simulink model "Copy_of_NDI"  (R2024b)
settings: Solver=ode4  StartTime=0  StopTime=100  FixedStep=fcs.Ts  RelTol=1e-3
PreLoadFcn:
  | FlightPhase = 'FallingLeaf';
  | % FlightPhase = 'InAir';
  | % FlightPhase = 'TVC_h10000V617alpha2';
  | run('PreLoadFcn.m')
values from neighbouring files (symbols this model uses):
  ControlAllocation = 1    [PreLoadFcn.m]    (also in RunThis_ChiaWei.m = 4; RunThis_LM.m = 4; RunThis_Shao.m; RunThis_james.m = 10)
  DUmax = IN_MAT(k+4,1:m)'    [LP_def.m]    (also in LP_lift.m; LP_sig.m; LP_thrust.m; PreLoadFcn.m = [Aactuator.right_aileron.RateLimitUpper Aactuator.left_ailer)
  DUmin = IN_MAT(k+5,1:m)'    [LP_def.m]    (also in LP_lift.m; LP_sig.m; LP_thrust.m; PreLoadFcn.m = [Aactuator.right_aileron.RateLimitLower Aactuator.left_ailer)
  g = [ 0  0  32.17 ]    [PreLoadFcn.m]
  hground = 0    [PreLoadFcn.m]
  m = m1-1    [CGIwrap.m]    (also in DAISY_CHAINING.m; DA_Allocation.m; LP_BasicSolution.m; LP_def.m)
  Mode_deflection_aileron = 1    [PreLoadFcn.m]    (also in RunThis_ChiaWei.m; RunThis_Shao.m = 0)
  Mode_deflection_elevator = 1    [PreLoadFcn.m]    (also in RunThis_ChiaWei.m; RunThis_Shao.m = 0)
  Mode_deflection_rudder = 1    [PreLoadFcn.m]    (also in RunThis_ChiaWei.m; RunThis_Shao.m = 0)
  Mode_deflection_TVC_y = 1    [PreLoadFcn.m]    (also in RunThis_ChiaWei.m; RunThis_Shao.m = 2)
  Mode_deflection_TVC_z = 1    [PreLoadFcn.m]    (also in RunThis_ChiaWei.m; RunThis_Shao.m = 0)
  N = IN_MAT(k+7:k+15,1:m)    [CGIwrap.m]    (also in DAISY_CHAINING.m; PreLoadFcn.m = [ 1      0     0.25; RunThis_ChiaWei.m = [ 1      0     0.25; RunThis_LM.m = [ 1      0     0.25)
  Ninv_2nozzle = inv(diag([  1/21.5  1/21.5  1/25  1/25  1/30  1/15  1/15  1/15  1/15 ]))    [PreLoadFcn.m]
  Ninv_no_nozzle = diag([    21.5    21.5    25    25    30    0     0     0     0  ])    [PreLoadFcn.m]
  state0 = [IC.npos IC.epos IC.alt IC.q0 IC.q1 IC.q2 IC.q3  IC.p IC.q IC.r IC.alpha IC.beta IC.mu IC.Vt IC.chi IC.gamma]    [PreLoadFcn.m]
  Umax_2nozzle = [Aactuator.right_aileron.AngleLimitUpper  Aactuator.left_aileron.AngleLimitUpper  Aactuator.right_elevator.AngleLimitUpper Aactuator.left_elevator.AngleLimitUpper  Aactuator.rudder.AngleLimitUpper                  Aactuator.TVC_ry.AngleLimitUpper    Aactuator.TVC_rz.AngleLimitUpper  Aactuator.TVC_ly.AngleLimitUpper    Aactuator.TVC_lz.AngleLimitUpper]    [PreLoadFcn.m]
  Umax_no_nozzle = [Aactuator.right_aileron.AngleLimitUpper  Aactuator.left_aileron.AngleLimitUpper  Aactuator.right_elevator.AngleLimitUpper Aactuator.left_elevator.AngleLimitUpper  Aactuator.rudder.AngleLimitUpper                    0 0 0 0]    [PreLoadFcn.m]
  Umin_2nozzle = [Aactuator.aileron.AngleLimitLower  Aactuator.aileron.AngleLimitLower  Aactuator.elevator.AngleLimitLower Aactuator.elevator.AngleLimitLower  Aactuator.rudder.AngleLimitLower                  Aactuator.TVC_ry.AngleLimitLower    Aactuator.TVC_rz.AngleLimitLower Aactuator.TVC_ly.AngleLimitLower    Aactuator.TVC_lz.AngleLimitLower]    [PreLoadFcn.m]
  Umin_no_nozzle = [Aactuator.right_aileron.AngleLimitLower  Aactuator.left_aileron.AngleLimitLower  Aactuator.right_elevator.AngleLimitLower Aactuator.left_elevator.AngleLimitLower  Aactuator.rudder.AngleLimitLower                    0 0 0 0]    [PreLoadFcn.m]
undefined symbols (not defined in the file or in its folder): Aactuator, ac, AeroCoeff, EngineTable, F, fcs, ft, IC, kg, LandingGear, Light, MIL, PIController, s, Sensor, sigbuilder_block, slug, sysID_DAQ, sysID_OBES, WMM2020
libraries: aerolibconvert2 x31, slpidlib x11, simulink x6, sharedutil x4, aerolibatmos2 x3, aerolibwind2 x3, aerolibbdyn x3, aerolibgravity2 x2, sharedtransform x1
(part 7 of 14)

== system Copy_of_NDI/F-16 Vehicle Systems Model/Vehicle/Propulsion(two_nozzles) ==
  note: Thrust Vector Nozzle Module 向量噴嘴模組
  note: Commands_TVC_ry_pitch_deg
      | Commands_TVC_rz_yaw_deg
      | Commands_TVC_ly_pitch_deg
      | Commands_TVC_lz_yaw_deg
  note: Inlet 進氣道
  note: 高度限制 0 ~ 50000 ft
      | 馬赫數限制 0 ~ 1 馬赫
  note: Thrust Vector Nozzle Module 向量噴嘴模組
  Bus Element In2 : Inport  PortName=fadec_cmd
  In Bus Element3 : Inport  PortName=fadec_cmd  Element=thrust
  In Bus Element1 : Inport  Port=2  PortName=EnvData  Element=Mach
  Bus Element In1 : Inport  Port=3  PortName=PlantData  Element=beta
  Bus Element In : Inport  Port=3  PortName=PlantData  Element=alpha
  In Bus Element : Inport  Port=3  PortName=PlantData  Element=altitude
  Actuators : Subsystem
  Actuators1 : Subsystem
  Add{,1..5} (6 alike) : Sum
  Afterburning Turbofan Jet Engine : Subsystem
  Bus Selector : BusSelector  OutputSignals=TVC_ly_pitch_deg,TVC_lz_yaw_deg
  Bus Selector1 : BusSelector  OutputSignals=TVC_ry_pitch_deg,TVC_rz_yaw_deg
  Cos : Trigonometry  Operator=cos
  Cos1 : Trigonometry  Operator=cos
  Gain1 : Gain  Gain=0.5
  IC1 : InitialCondition  Commented=through  Value=IC.thrust_lbf
  Left Thrust Vector Nozzle ZY : Subsystem
  Mux2 : Mux  Inputs=6
  Product : Product  Inputs=3
  Right Thrust Vector Nozzle ZY : Subsystem
  nozzle position1 : Constant  Value=ac.lt1
  nozzle position2 : Constant  Value=ac.mt
  nozzle position3 : Constant  Value=ac.lt1
  nozzle position4 : Constant  Value=ac.mt
  r2d1 : Gain  Gain=-1  SaturateOnIntegerOverflow=on  OutDataTypeStr=Inherit: Same as input  ParamDataTypeStr=Inherit: Same as input
  FM : Outport
  Bus Element Out : Outport  Port=2  PortName=ActSensor_Out  Element=TVC_ry_pitch_deg
  Bus Element Out1 : Outport  Port=2  PortName=ActSensor_Out  Element=TVC_rz_yaw_deg
  Bus Element Out2 : Outport  Port=2  PortName=ActSensor_Out  Element=TVC_ly_pitch_deg
  Bus Element Out3 : Outport  Port=2  PortName=ActSensor_Out  Element=TVC_lz_yaw_deg
  Bus Element Out4 : Outport  Port=3  PortName=PropData  Element=T
  Bus Element Out5 : Outport  Port=3  PortName=PropData  Element=engine_state
  Bus Element Out15 : Outport  Port=3  PortName=PropData  Element=Tx
  Bus Element Out16 : Outport  Port=3  PortName=PropData  Element=Ty
  Bus Element Out17 : Outport  Port=3  PortName=PropData  Element=Tz
  wires:
  nozzle position1/1 -> Right Thrust Vector Nozzle ZY/3(" lt")
  Product/1 -> Afterburning Turbofan Jet Engine/1(Mach)
  r2d1/1 -> Afterburning Turbofan Jet Engine/2(H (ft))
  Cos/1 -> Product/2
  Bus Element In1/1 -> Cos1/1  "beta (rad)"
  In Bus Element1/1 -> Product/1
  Cos1/1 -> Product/3
  Bus Element In/1 -> Cos/1  "alpha (rad)"
  In Bus Element/1 -> r2d1/1
  Bus Element In2/1 -> Actuators1/1(Commands), Actuators/1(Commands)
  Right Thrust Vector Nozzle ZY/1(Trx) -> Add/1
  Right Thrust Vector Nozzle ZY/2(Try) -> Add1/1
  Right Thrust Vector Nozzle ZY/3(Trz) -> Add2/1
  nozzle position2/1 -> Right Thrust Vector Nozzle ZY/4(" mt")
  IC1/1 -> Gain1/1, Bus Element Out4/1
  Afterburning Turbofan Jet Engine/1(T (lbf)) -> IC1/1  "thrust"
  Afterburning Turbofan Jet Engine/2(engine_state) -> Bus Element Out5/1
  In Bus Element3/1 -> Afterburning Turbofan Jet Engine/3(Tc (lbf))  "Commands_Tc"
  Gain1/1 -> Left Thrust Vector Nozzle ZY/1(T), Right Thrust Vector Nozzle ZY/1(T)
  Right Thrust Vector Nozzle ZY/4(Mrx) -> Add3/1
  Right Thrust Vector Nozzle ZY/5(Mry) -> Add4/1
  Right Thrust Vector Nozzle ZY/6(Mrz) -> Add5/1
  nozzle position3/1 -> Left Thrust Vector Nozzle ZY/3(" lt")
  nozzle position4/1 -> Left Thrust Vector Nozzle ZY/4(" mt")
  Actuators1/1(ActPositions) -> Left Thrust Vector Nozzle ZY/2(Actuator (deg))
  Left Thrust Vector Nozzle ZY/1(Tlx) -> Add/2
  Left Thrust Vector Nozzle ZY/2(Tly) -> Add1/2
  Left Thrust Vector Nozzle ZY/3(Tlz) -> Add2/2
  Left Thrust Vector Nozzle ZY/4(Mlx) -> Add3/2
  Left Thrust Vector Nozzle ZY/5(Mly) -> Add4/2
  Left Thrust Vector Nozzle ZY/6(Mlz) -> Add5/2
  Add/1 -> Bus Element Out15/1, Mux2/1
  Add1/1 -> Bus Element Out16/1, Mux2/2
  Add2/1 -> Mux2/3, Bus Element Out17/1
  Add3/1 -> Mux2/4
  Add4/1 -> Mux2/5
  Add5/1 -> Mux2/6
  Mux2/1 -> FM/1
  Actuators/2(ActSensor_Out) -> Bus Selector1/1
  Actuators1/2(ActSensor_Out) -> Bus Selector/1
  Bus Selector/1 -> Bus Element Out2/1  "<TVC_ly_pitch_deg>"
  Bus Selector/2 -> Bus Element Out3/1  "<TVC_lz_yaw_deg>"
  Bus Selector1/1 -> Bus Element Out/1  "<TVC_ry_pitch_deg>"
  Bus Selector1/2 -> Bus Element Out1/1  "<TVC_rz_yaw_deg>"
  Actuators/1(ActPositions) -> Right Thrust Vector Nozzle ZY/2(Actuator (deg))

== system Copy_of_NDI/F-16 Vehicle Systems Model/pqr NDI Controller/Control Allocation ==
  note: 多級偽逆法
  note: 108、109年度學合案
      | 2019張舜淵論文配置法
  note: 最小雷達散射截面積
  note: 最小控制面偏轉量
  note: 最小向量推力
  note: 最大升力
  note: 線性規劃法基礎解
  note: 管理方案三：廣義逆類配置法
  note: 管理方案二：基於期望力矩
  note: 直接幾何法
  note: 多級偽逆法
  note: 串接鏈配置法
  note: 加權偽逆法
  IN_MAT1 : Inport
  alpha (deg) : Inport  Port=2
  Vt (ft/s) : Inport  Port=3
  altitude (ft) : Inport  Port=4
  y_bar : Inport  Port=5
  g1 : Inport  Port=6
  N : Inport  Port=7
  Abs : Abs  SaturateOnIntegerOverflow=off
  Abs1 : Abs  SaturateOnIntegerOverflow=off
  Abs2 : Abs  SaturateOnIntegerOverflow=off
  CGIwrap : Subsystem  TreatAsAtomicUnit=on
  CGIwrap1 : Subsystem  TreatAsAtomicUnit=on
  Chart : Stateflow chart  TreatAsAtomicUnit=on  SystemSampleTime=fcs.Ts
      settings: PortSchema="{\"entries\":[{\"content\":{\"sides\":[{\"content\":{\"connectorIds\":[\"In6\",\"In1\",\"In2\",\"In4\",\"In3\",\"In5\"]},\"type\":\"ConnectorPlacement.EquallySpacedRectSide\",\"uuid\":\"6d076ae3-a9f2-4680-9177-aea4e2fc761d\"},{\"content\":{\"connectorIds\":[\"Out1\"],\"side\":\"RIGHT\"},\"type\":\"ConnectorPlacement.EquallySpacedRectSide\",\"uuid\":\"02bbf86f-ce68-419e-b070-bdc8bcbcb5dc\"},{\"content\":{\"connectorIds\":[],\"side\":\"TOP\"},\"type\":\"ConnectorPlacement.EquallySpacedRectSide\",\"uuid\":\"3dbba490-ab37-41e3-b3e5-776a7fc0e7cf\"}]},\"type\":\"ConnectorPlacement.EquallySpacedConnector\",\"uuid\":\"e8ffa1d9-13bd-4b1f-b66c-de77a24e235e\"}],\"packageUris\":[\"http://schema.mathworks.com/mf0/Connector/19700101\"],\"version\":\"1.0\"}"
  Constant : Constant  Value=0
  ControlAllocation : Constant  Value=ControlAllocation
  DAISY_CHAINING : Subsystem  TreatAsAtomicUnit=on
  DA_Allocation : Subsystem  TreatAsAtomicUnit=on
  Discrete Derivative : simulink/Discrete/Discrete Derivative  gainval=1.0  ICPrevScaledInput=0.0  OutMin=[]  OutMax=[]  OutDataType=fixdt(1, 16)  OutScaling=2^-10  DoSatur=off
  Discrete Derivative1 : simulink/Discrete/Discrete Derivative  gainval=1.0  ICPrevScaledInput=0.0  OutMin=[]  OutMax=[]  OutDataType=fixdt(1, 16)  OutScaling=2^-10  DoSatur=off
  IC : InitialCondition  Value=0
  IC1 : InitialCondition  Value=0
  IC2 : InitialCondition  Value=[0 0 0 0 0 0 0 0 0]
  If : If  IfExpression=u1 == 1  ElseIfExpressions=u1 == 2,u1 == 3,u1 == 4,u1 == 5,u1==6,u1==7,u1==8,u1==9,u1==10,u1==11,u1==12
  LP_BasicSolution : Subsystem  TreatAsAtomicUnit=on
  LP_def : Subsystem  TreatAsAtomicUnit=on
  LP_lift : Subsystem  TreatAsAtomicUnit=on
  LP_sig : Subsystem  TreatAsAtomicUnit=on
  LP_thrust : Subsystem  TreatAsAtomicUnit=on
  Manual Switch : ManualSwitch  CurrentSetting=0
  Merge1 : Merge  Inputs=13
  Pseudo_inverses_ShunYuanChang2019 : Subsystem  TreatAsAtomicUnit=on
  To Workspace : ToWorkspace  VariableName=u  SaveFormat=Timeseries  SampleTime=-1
  To Workspace1 : ToWorkspace  VariableName=altitude_dot  SaveFormat=Timeseries  SampleTime=-1
  To Workspace2 : ToWorkspace  VariableName=Vt_dot  SaveFormat=Timeseries  SampleTime=-1
  Weighted_Pseudo_inverses : Subsystem  TreatAsAtomicUnit=on
  control_management2 : Subsystem  TreatAsAtomicUnit=on
  control_management3 : Subsystem  TreatAsAtomicUnit=on
  Du : Outport
  wires:
  DAISY_CHAINING/1(Out1) -> Merge1/2
  Weighted_Pseudo_inverses/1(Out1) -> Merge1/1
  IN_MAT1/1 -> LP_thrust/1(IN_MAT), LP_sig/1(IN_MAT), CGIwrap1/1(IN_MAT), LP_def/1(IN_MAT), LP_lift/1(IN_MAT), control_management2/1(IN_MAT), DA_Allocation/1(IN_MAT), CGIwrap/1(IN_MAT), Weighted_Pseudo_inverses/1(IN_MAT), DAISY_CHAINING/1(IN_MAT), control_management3/1(IN_MAT), LP_BasicSolution/1(IN_MAT)
  Chart/1(CA) -> Manual Switch/1
  ControlAllocation/1 -> Manual Switch/2
  LP_thrust/1(Out1) -> Merge1/9
  LP_def/1(Out1) -> Merge1/10
  LP_sig/1(Out1) -> Merge1/11
  alpha (deg)/1 -> Chart/1(alpha)
  altitude (ft)/1 -> Abs/1
  Abs/1 -> Chart/3(altitude), Discrete Derivative1/1
  Discrete Derivative/1 -> Abs1/1
  Discrete Derivative1/1 -> Abs2/1
  Vt (ft/s)/1 -> Chart/2(Vt), Discrete Derivative/1
  IC/1 -> Chart/5(altitude_dot), To Workspace1/1
  Abs2/1 -> IC/1
  Abs1/1 -> IC1/1
  IC1/1 -> Chart/4(Vt_dot), To Workspace2/1
  Pseudo_inverses_ShunYuanChang2019/1(Output) -> Merge1/12
  y_bar/1 -> Pseudo_inverses_ShunYuanChang2019/1(y_bar)
  g1/1 -> Pseudo_inverses_ShunYuanChang2019/2(g1)
  N/1 -> Pseudo_inverses_ShunYuanChang2019/3(N)
  Constant/1 -> Chart/6(switchhh)
  LP_lift/1(Out1) -> Merge1/8
  IC2/1 -> Du/1
  Merge1/1 -> IC2/1
  Manual Switch/1 -> If/1, To Workspace/1
  CGIwrap1/1(Out1) -> Merge1/13
  DA_Allocation/1(Out1) -> Merge1/4
  CGIwrap/1(Out1) -> Merge1/3
  LP_BasicSolution/1(Out1) -> Merge1/7
  control_management3/1(Out1) -> Merge1/6
  control_management2/1(Out1) -> Merge1/5
  If/1 -> Weighted_Pseudo_inverses/Action
  If/2 -> DAISY_CHAINING/Action
  If/3 -> CGIwrap/Action
  If/4 -> DA_Allocation/Action
  If/5 -> control_management2/Action
  If/6 -> control_management3/Action
  If/7 -> LP_BasicSolution/Action
  If/8 -> LP_lift/Action
  If/9 -> LP_thrust/Action
  If/10 -> LP_def/Action
  If/11 -> LP_sig/Action
  If/12 -> Pseudo_inverses_ShunYuanChang2019/Action
  If/13 -> CGIwrap1/Action

== system Copy_of_NDI/F-16 Vehicle Systems Model/pqr NDI Controller/MakeINMAT ==
  note: 飛控系統的取樣時間(秒)
  note: 控制配置的權重矩陣 $N^{-1}$
      | (定義於 PreLoadFcn.m)
  note: 下標1表示在列後面擴增
      | 下標2表示在行後面擴增
  f1 : Inport
  g1 : Inport  Port=2
  In3 : Inport  Port=3
  Constant1 : Constant  Value=[0;0;0;0;0]
  Constant10 : Constant  Value=Umin_no_nozzle
  Constant2 : Constant  Value=Umax_2nozzle
  Constant3 : Constant  Value=Umin_2nozzle
  Constant4 : Constant  Value=[1 1 1 1 1 1 1 1 1]
  Constant5 : Constant  Value=fcs.Ts
  Constant6 : Constant  Value=DUmax
  Constant7 : Constant  Value=[0;0;0;0;0;0;0;0;0]
  Constant8 : Constant  Value=DUmin
  Constant9 : Constant  Value=Umax_no_nozzle
  Manual Switch : ManualSwitch
  Manual Switch1 : ManualSwitch
  Manual Switch2 : ManualSwitch
  Matrix Concatenate{,2,4,6} (4 alike) : Concatenate  Mode=Multidimensional array  ConcatenateDimension=2
  Matrix Concatenate3 : Concatenate  NumInputs=5  Mode=Multidimensional array
  Matrix Concatenate5 : Concatenate  NumInputs=4  Mode=Multidimensional array
  Signal Specification : SignalSpecification  Dimensions=[3 1]
  Signal Specification{1..2,4..9} (8 alike) : SignalSpecification  Dimensions=[1,9]
  Signal Specification3 : SignalSpecification  Dimensions=[3 9]
  To Workspace2 : ToWorkspace  VariableName=B_matrix  SaveFormat=Timeseries  SampleTime=-1
  inverse of weighting matrix N : Constant  Value=Ninv_2nozzle
  inverse of weighting matrix N1 : Constant  Value=Ninv_no_nozzle
  IN_MAT : Outport
  wires:
  Matrix Concatenate6/1 -> Matrix Concatenate5/4
  Matrix Concatenate3/1 -> Matrix Concatenate4/1
  Signal Specification3/1 -> Matrix Concatenate/1
  Manual Switch1/1 -> Matrix Concatenate3/2
  Matrix Concatenate4/1 -> Matrix Concatenate5/3
  Matrix Concatenate/1 -> Matrix Concatenate5/1
  Signal Specification/1 -> Matrix Concatenate/2
  Manual Switch/1 -> Matrix Concatenate3/1
  Matrix Concatenate5/1 -> IN_MAT/1
  f1/1 -> Signal Specification/1
  g1/1 -> To Workspace2/1, Signal Specification3/1
  Constant4/1 -> Signal Specification4/1
  Signal Specification4/1 -> Matrix Concatenate3/5
  Constant1/1 -> Matrix Concatenate4/2
  In3/1 -> Signal Specification5/1
  Signal Specification5/1 -> Matrix Concatenate2/1
  Constant5/1 -> Matrix Concatenate2/2
  Matrix Concatenate2/1 -> Matrix Concatenate5/2
  Signal Specification6/1 -> Matrix Concatenate3/3
  Signal Specification7/1 -> Matrix Concatenate3/4
  Constant6/1 -> Signal Specification6/1  "Umax"
  Constant8/1 -> Signal Specification7/1  "Umax"
  Constant3/1 -> Signal Specification2/1  "Umin"
  Constant2/1 -> Signal Specification1/1  "Umax"
  Signal Specification1/1 -> Manual Switch/1
  Signal Specification2/1 -> Manual Switch1/1
  Signal Specification8/1 -> Manual Switch/2
  Constant9/1 -> Signal Specification8/1  "Umax"
  Signal Specification9/1 -> Manual Switch1/2
  Constant10/1 -> Signal Specification9/1  "Umin"
  Constant7/1 -> Matrix Concatenate6/2
  inverse of weighting matrix N/1 -> Manual Switch2/1
  inverse of weighting matrix N1/1 -> Manual Switch2/2
  Manual Switch2/1 -> Matrix Concatenate6/1

== system Copy_of_NDI/F-16 Vehicle Systems Model/pqr NDI Controller/Mode_deflection ==
  note: 偏轉模式： 0=傳統左右副翼差動
      | 1=左右副翼獨立偏轉
      | 其它=左右副翼獨立偏轉
  note: 偏轉模式： 0=傳統左右升降舵同動
      | 1=左右升降舵獨立偏轉
      | 其它=左右升降舵獨立偏轉
  note: 偏轉模式： 0=傳統左右方向舵同動
      | 1=左右方向舵獨立偏轉
      | 2=左右方向舵差動(產生減速效果)
      | 其它=左右方向舵獨立偏轉
  note: 偏轉模式： 0=傳統左右向量噴嘴固定不動
      | 1=左右向量噴嘴左右獨立偏轉
      | 2=左右向量噴嘴左右同動
      | 其它=左右向量噴嘴左右獨立偏轉
  note: 偏轉模式： 0=傳統左右向量噴嘴固定不動
      | 1=左右向量噴嘴上下獨立偏轉
      | 2=左右向量噴嘴上下同動(產生俯仰)
      | 3=左右向量噴嘴上下差動(產生滾轉)
      | 其它=左右向量噴嘴上下獨立偏轉
  dra : Inport
  dla : Inport  Port=2
  dre : Inport  Port=3
  dle : Inport  Port=4
  drr : Inport  Port=5
  dlr : Inport  Port=6
  dry : Inport  Port=7
  drz : Inport  Port=8
  dly : Inport  Port=9
  dlz : Inport  Port=10
  Constant{,3,7,10} (4 alike) : Constant  Value=0
  Constant1 : Constant  Value=Mode_deflection_aileron
  Constant2 : Constant  Value=Mode_deflection_elevator
  Constant4 : Constant  Value=Mode_deflection_TVC_y
  Constant5 : Constant  Value=Mode_deflection_rudder
  Constant6 : Constant  Value=Mode_deflection_TVC_y
  Constant8 : Constant  Value=Mode_deflection_TVC_z
  Constant9 : Constant  Value=Mode_deflection_TVC_z
  Gain : Gain  Gain=-1
  Gain1 : Gain  Gain=-1
  Gain2 : Gain  Gain=-1
  Multiport Switch : MultiPortSwitch  DataPortOrder=Zero-based contiguous  Inputs=2  zeroidx=on  SaturateOnIntegerOverflow=off  InputSameDT=off
  Multiport Switch1 : MultiPortSwitch  DataPortOrder=Zero-based contiguous  Inputs=2  zeroidx=on  SaturateOnIntegerOverflow=off  InputSameDT=off
  Multiport Switch2 : MultiPortSwitch  DataPortOrder=Zero-based contiguous  DataPortForDefault=Additional data port  zeroidx=on  SaturateOnIntegerOverflow=off  InputSameDT=off
  Multiport Switch3 : MultiPortSwitch  DataPortOrder=Zero-based contiguous  Inputs=4  DataPortForDefault=Additional data port  zeroidx=on  SaturateOnIntegerOverflow=off  InputSameDT=off
  Multiport Switch4 : MultiPortSwitch  DataPortOrder=Zero-based contiguous  DataPortForDefault=Additional data port  zeroidx=on  SaturateOnIntegerOverflow=off  InputSameDT=off
  Multiport Switch5 : MultiPortSwitch  DataPortOrder=Zero-based contiguous  Inputs=4  DataPortForDefault=Additional data port  zeroidx=on  SaturateOnIntegerOverflow=off  InputSameDT=off
  Multiport Switch6 : MultiPortSwitch  DataPortOrder=Zero-based contiguous  DataPortForDefault=Additional data port  zeroidx=on  SaturateOnIntegerOverflow=off  InputSameDT=off
  right_aileron : Outport  VectorParamsAs1DForOutWhenUnconnected=off
  left_aileron : Outport  Port=2  VectorParamsAs1DForOutWhenUnconnected=off
  right_elevator : Outport  Port=3  VectorParamsAs1DForOutWhenUnconnected=off
  left_elevator : Outport  Port=4  VectorParamsAs1DForOutWhenUnconnected=off
  rudder : Outport  Port=5  VectorParamsAs1DForOutWhenUnconnected=off
  left_rudder : Outport  Port=6  VectorParamsAs1DForOutWhenUnconnected=off
  "TVC_ry " : Outport  Port=7  VectorParamsAs1DForOutWhenUnconnected=off
  TVC_rz : Outport  Port=8  VectorParamsAs1DForOutWhenUnconnected=off
  "TVC_ly " : Outport  Port=9  VectorParamsAs1DForOutWhenUnconnected=off
  "TVC_lz " : Outport  Port=10  VectorParamsAs1DForOutWhenUnconnected=off
  wires:
  Gain2/1 -> Multiport Switch3/5
  Gain1/1 -> Multiport Switch4/4
  Multiport Switch4/1 -> left_rudder/1
  Multiport Switch2/1 -> "TVC_lz "/1
  Constant3/1 -> Multiport Switch2/2
  drz/1 -> Multiport Switch6/3, Multiport Switch6/4, Multiport Switch6/5, Multiport Switch2/4
  Constant10/1 -> Multiport Switch6/2
  Multiport Switch6/1 -> TVC_rz/1
  Constant8/1 -> Multiport Switch2/1
  dlz/1 -> Multiport Switch2/3, Multiport Switch2/5
  Constant9/1 -> Multiport Switch6/1
  Multiport Switch5/1 -> "TVC_ry "/1
  Constant7/1 -> Multiport Switch5/2
  Constant6/1 -> Multiport Switch5/1
  Constant/1 -> Multiport Switch3/2
  dly/1 -> Multiport Switch3/6, Multiport Switch3/3
  Multiport Switch/1 -> left_aileron/1
  dre/1 -> right_elevator/1, Multiport Switch1/2
  dle/1 -> Multiport Switch1/3
  Multiport Switch1/1 -> left_elevator/1
  dla/1 -> Multiport Switch/3
  drr/1 -> Multiport Switch4/2, Gain1/1, rudder/1
  dry/1 -> Gain2/1, Multiport Switch3/4, Multiport Switch5/6, Multiport Switch5/5, Multiport Switch5/4, Multiport Switch5/3
  Constant5/1 -> Multiport Switch4/1
  dra/1 -> right_aileron/1, Gain/1
  Constant2/1 -> Multiport Switch1/1
  Constant4/1 -> Multiport Switch3/1
  Gain/1 -> Multiport Switch/2
  Constant1/1 -> Multiport Switch/1
  dlr/1 -> Multiport Switch4/3, Multiport Switch4/5
  Multiport Switch3/1 -> "TVC_ly "/1

== system Copy_of_NDI/F-16 Vehicle Systems Model/pqr NDI Controller/control matrix g1 ==
  note: m
      | ix
      | iy
      | iz
      | ixy
      | ixz
      | iyz
  note: 1  gp_dra1
      |     gp_dla1
      |     gp_dre1
      |     gp_dle1
      |     gp_dr1
      |     gp_dra2
      |     gp_dla2
      |     gp_dre2
      |     gp_dle2
      |     gp_dr2
      |
      | 11 gq_dra
      |      gq_dla
      |      gq_dre
      |      gq_dle
      |
      | 15 gr_dra1
      |      gr_dla1
      |      gr_dre1
      |      gr_dle1
      |      gr_dr1
      |      gr_dra2
      |      gr_dla2
      |      gr_dre2
      |      gr_dle2
      |      gr_dr2
  note: $g_1 {\left({\overset{-}{x} }_1 \right)}={\left[\begin{array}{ccccccccc} g_{p_{\delta_{ra} } } & g_{p_{\delta_{la} } } & g_{p_{\delta_{re} } } & g_{p_{\delta_{le} } } & g_{p_{\delta_r } } & g_{p_{\delta_{ry} } } & g_{p_{\delta_{rz} } } & g_{p_{\delta_{ly} } } & g_{p_{\delta_{lz} } } \\ g_{q_{\delta_{ra} } } & g_{q_{\delta_{la} } } & g_{q_{\delta_{re} } } & g_{q_{\delta_{le} } } & 0 & g_{q_{\delta_{ry} } } & 0 & g_{q_{\delta_{ly} } } & 0 \\ g_{r_{\delta_{ra} } } & g_{r_{\delta_{la} } } & g_{r_{\delta_{re} } } & g_{r_{\delta_{le} } } & g_{r_{\delta_r } } & g_{r_{\delta_{ry} } } & g_{r_{\delta_{rz} } } & g_{r_{\delta_{ly} } } & g_{r_{\delta_{lz} } } \end{array}\right]}$
  coef g : Inport
  Thrust T : Inport  Port=2
  Engine nozzle after of c.g.1 : Constant  Value=ac.lt1
  Engine nozzle after of c.g.2 : Constant  Value=ac.mt
  Gain : Gain  Gain=1/2
  Ix(slug*ft^2) : Constant  Value=ac.Ix
  Ixy(slug*ft^2) : Constant  Value=ac.Ixy
  Ixz(slug*ft^2) : Constant  Value=ac.Ixz
  Iy(slug*ft^2) : Constant  Value=ac.Iy
  Iyz(slug*ft^2) : Constant  Value=ac.Iyz
  Iz(slug*ft^2) : Constant  Value=ac.Iz
  Matrix Concatenate : Concatenate  NumInputs=3  Mode=Multidimensional array
  Mux : Mux  Inputs=7
  "Pitching " : Subsystem
  "Rolling " : Subsystem
  "Yawing " : Subsystem
  m(slugs) : Constant  Value=ac.m
  g1 : Outport  VectorParamsAs1DForOutWhenUnconnected=off
  wires:
  "Yawing "/1(g1 Row3) -> Matrix Concatenate/3
  "Pitching "/1(g1 Row2) -> Matrix Concatenate/2
  "Rolling "/1(g1 Row1) -> Matrix Concatenate/1
  Mux/1 -> "Rolling "/2(inertia), "Pitching "/2(inertia), "Yawing "/2(inertia)
  coef g/1 -> "Yawing "/1(control_g), "Pitching "/1(control_g), "Rolling "/1(control_g)
  Thrust T/1 -> Gain/1
  Engine nozzle after of c.g.1/1 -> "Yawing "/4("lt1 "), "Pitching "/4(lt1), "Rolling "/4(lt1)
  Iyz(slug*ft^2)/1 -> Mux/7
  Ix(slug*ft^2)/1 -> Mux/2
  Iy(slug*ft^2)/1 -> Mux/3
  Ixy(slug*ft^2)/1 -> Mux/5
  Ixz(slug*ft^2)/1 -> Mux/6
  Iz(slug*ft^2)/1 -> Mux/4
  m(slugs)/1 -> Mux/1
  Matrix Concatenate/1 -> g1/1
  Engine nozzle after of c.g.2/1 -> "Rolling "/5(mt), "Pitching "/5(mt), "Yawing "/5(mt)
  Gain/1 -> "Rolling "/3(Thrust), "Pitching "/3(Thrust), "Yawing "/3(Thrust)

== system Copy_of_NDI/F-16 Vehicle Systems Model/sysID_Onboard_Excitation_System/Mode_deflection ==
  note: 偏轉模式： 0=傳統左右副翼差動
      | 1=左右副翼獨立偏轉
      | 其它=左右副翼獨立偏轉
  note: 偏轉模式： 0=傳統左右升降舵同動
      | 1=左右升降舵獨立偏轉
      | 其它=左右升降舵獨立偏轉
  note: 偏轉模式： 0=傳統左右方向舵同動
      | 1=左右方向舵獨立偏轉
      | 2=左右方向舵差動(產生減速效果)
      | 其它=左右方向舵獨立偏轉
  note: 偏轉模式： 0=傳統左右向量噴嘴固定不動
      | 1=左右向量噴嘴左右獨立偏轉
      | 2=左右向量噴嘴左右同動
      | 其它=左右向量噴嘴左右獨立偏轉
  note: 偏轉模式： 0=傳統左右向量噴嘴固定不動
      | 1=左右向量噴嘴上下獨立偏轉
      | 2=左右向量噴嘴上下同動(產生俯仰)
      | 3=左右向量噴嘴上下差動(產生滾轉)
      | 其它=左右向量噴嘴上下獨立偏轉
  dra : Inport
  dla : Inport  Port=2
  dre : Inport  Port=3
  dle : Inport  Port=4
  drr : Inport  Port=5
  dlr : Inport  Port=6
  dry : Inport  Port=7
  drz : Inport  Port=8
  dly : Inport  Port=9
  dlz : Inport  Port=10
  Constant{,3,7,10} (4 alike) : Constant  Value=0
  Constant1 : Constant  Value=Mode_deflection_aileron
  Constant2 : Constant  Value=Mode_deflection_elevator
  Constant4 : Constant  Value=Mode_deflection_TVC_y
  Constant5 : Constant  Value=Mode_deflection_rudder
  Constant6 : Constant  Value=Mode_deflection_TVC_y
  Constant8 : Constant  Value=Mode_deflection_TVC_z
  Constant9 : Constant  Value=Mode_deflection_TVC_z
  Gain : Gain  Gain=-1
  Gain1 : Gain  Gain=-1
  Gain2 : Gain  Gain=-1
  Multiport Switch : MultiPortSwitch  DataPortOrder=Zero-based contiguous  Inputs=2  zeroidx=on  SaturateOnIntegerOverflow=off  InputSameDT=off
  Multiport Switch1 : MultiPortSwitch  DataPortOrder=Zero-based contiguous  Inputs=2  zeroidx=on  SaturateOnIntegerOverflow=off  InputSameDT=off
  Multiport Switch2 : MultiPortSwitch  DataPortOrder=Zero-based contiguous  DataPortForDefault=Additional data port  zeroidx=on  SaturateOnIntegerOverflow=off  InputSameDT=off
  Multiport Switch3 : MultiPortSwitch  DataPortOrder=Zero-based contiguous  Inputs=4  DataPortForDefault=Additional data port  zeroidx=on  SaturateOnIntegerOverflow=off  InputSameDT=off
  Multiport Switch4 : MultiPortSwitch  DataPortOrder=Zero-based contiguous  DataPortForDefault=Additional data port  zeroidx=on  SaturateOnIntegerOverflow=off  InputSameDT=off
  Multiport Switch5 : MultiPortSwitch  DataPortOrder=Zero-based contiguous  Inputs=4  DataPortForDefault=Additional data port  zeroidx=on  SaturateOnIntegerOverflow=off  InputSameDT=off
  Multiport Switch6 : MultiPortSwitch  DataPortOrder=Zero-based contiguous  DataPortForDefault=Additional data port  zeroidx=on  SaturateOnIntegerOverflow=off  InputSameDT=off
  right_aileron : Outport  VectorParamsAs1DForOutWhenUnconnected=off
  left_aileron : Outport  Port=2  VectorParamsAs1DForOutWhenUnconnected=off
  right_elevator : Outport  Port=3  VectorParamsAs1DForOutWhenUnconnected=off
  left_elevator : Outport  Port=4  VectorParamsAs1DForOutWhenUnconnected=off
  rudder : Outport  Port=5  VectorParamsAs1DForOutWhenUnconnected=off
  left_rudder : Outport  Port=6  VectorParamsAs1DForOutWhenUnconnected=off
  "TVC_ry " : Outport  Port=7  VectorParamsAs1DForOutWhenUnconnected=off
  TVC_rz : Outport  Port=8  VectorParamsAs1DForOutWhenUnconnected=off
  "TVC_ly " : Outport  Port=9  VectorParamsAs1DForOutWhenUnconnected=off
  "TVC_lz " : Outport  Port=10  VectorParamsAs1DForOutWhenUnconnected=off
  wires:
  Gain2/1 -> Multiport Switch3/5
  Gain1/1 -> Multiport Switch4/4
  Multiport Switch4/1 -> left_rudder/1
  Multiport Switch2/1 -> "TVC_lz "/1
  Constant3/1 -> Multiport Switch2/2
  drz/1 -> Multiport Switch6/3, Multiport Switch6/4, Multiport Switch6/5, Multiport Switch2/4
  Constant10/1 -> Multiport Switch6/2
  Multiport Switch6/1 -> TVC_rz/1
  Constant8/1 -> Multiport Switch2/1
  dlz/1 -> Multiport Switch2/3, Multiport Switch2/5
  Constant9/1 -> Multiport Switch6/1
  Multiport Switch5/1 -> "TVC_ry "/1
  Constant7/1 -> Multiport Switch5/2
  Constant6/1 -> Multiport Switch5/1
  Constant/1 -> Multiport Switch3/2
  dly/1 -> Multiport Switch3/6, Multiport Switch3/3
  Multiport Switch/1 -> left_aileron/1
  dre/1 -> right_elevator/1, Multiport Switch1/2
  dle/1 -> Multiport Switch1/3
  Multiport Switch1/1 -> left_elevator/1
  dla/1 -> Multiport Switch/3
  drr/1 -> Multiport Switch4/2, Gain1/1, rudder/1
  dry/1 -> Gain2/1, Multiport Switch3/4, Multiport Switch5/6, Multiport Switch5/5, Multiport Switch5/4, Multiport Switch5/3
  Constant5/1 -> Multiport Switch4/1
  dra/1 -> right_aileron/1, Gain/1
  Constant2/1 -> Multiport Switch1/1
  Constant4/1 -> Multiport Switch3/1
  Gain/1 -> Multiport Switch/2
  Constant1/1 -> Multiport Switch/1
  dlr/1 -> Multiport Switch4/3, Multiport Switch4/5
  Multiport Switch3/1 -> "TVC_ly "/1

== system Copy_of_NDI/F-16 Vehicle Systems Model/sysID_Onboard_Excitation_System/signal generator ==
  note: ROM記憶體的指標(Pointer)
  note: 唯讀記憶體，裡面存放波形
  isTurnOn : Inport
  Enable : Inport  Port=2
  sysID_isDone : Inport  Port=3
  Constant1 : Constant  Value=sysID_OBES.TVC_ry.amplitude
  Index Vector : MultiPortSwitch  Inputs=1  SaturateOnIntegerOverflow=off  InputSameDT=off
  Logical Operator1 : Logic  AllPortsSameDT=off  OutDataTypeStr=boolean
  Logical Operator3 : Logic  Operator=NOT  AllPortsSameDT=off  OutDataTypeStr=boolean
  Logical Operator4 : Logic  AllPortsSameDT=off  OutDataTypeStr=boolean
  Pause Counter : Subsystem  TreatAsAtomicUnit=on
  Product : Product
  ROM : Constant  Value=sysID_OBES.TVC_ry.wave
  TVC_ry_delay : Delay  DelayLength=sysID_OBES.TVC_ry.delay/sysID_OBES.Ts  SampleTime=sysID_OBES.Ts
  signal : Outport  OutputWhenDisabled=reset  InitialOutput=0
  isDone : Outport  Port=2
  wires:
  ROM/1 -> Index Vector/2
  Pause Counter/1(CountValue) -> Index Vector/1  "Pointer"
  Pause Counter/2(isCountDone) -> isDone/1
  Constant1/1 -> Product/1
  Index Vector/1 -> Product/2
  Product/1 -> signal/1
  Logical Operator3/1 -> Logical Operator4/2
  sysID_isDone/1 -> Logical Operator3/1  "isDone"
  TVC_ry_delay/1 -> Logical Operator4/1
  Enable/1 -> TVC_ry_delay/1  "isEnable"
  isTurnOn/1 -> Logical Operator1/1  "isTurnOn"
  Logical Operator4/1 -> Logical Operator1/2  "enableSignal"
  Logical Operator1/1 -> Pause Counter/Enable

== system Copy_of_NDI/F-16 Vehicle Systems Model/sysID_Onboard_Excitation_System/signal generator1 ==
  note: ROM記憶體的指標(Pointer)
  note: 唯讀記憶體，裡面存放波形
  isTurnOn : Inport
  Enable : Inport  Port=2
  sysID_isDone : Inport  Port=3
  Constant1 : Constant  Value=sysID_OBES.TVC_rz.amplitude
  Index Vector : MultiPortSwitch  Inputs=1  SaturateOnIntegerOverflow=off  InputSameDT=off
  Logical Operator1 : Logic  AllPortsSameDT=off  OutDataTypeStr=boolean
  Logical Operator3 : Logic  Operator=NOT  AllPortsSameDT=off  OutDataTypeStr=boolean
  Logical Operator4 : Logic  AllPortsSameDT=off  OutDataTypeStr=boolean
  Pause Counter : Subsystem  TreatAsAtomicUnit=on
  Product : Product
  ROM : Constant  Value=sysID_OBES.TVC_rz.wave
  TVC_rz_delay : Delay  DelayLength=sysID_OBES.TVC_rz.delay/sysID_OBES.Ts  SampleTime=sysID_OBES.Ts
  signal : Outport  OutputWhenDisabled=reset  InitialOutput=0
  isDone : Outport  Port=2
  wires:
  ROM/1 -> Index Vector/2
  Pause Counter/1(CountValue) -> Index Vector/1  "Pointer"
  Pause Counter/2(isCountDone) -> isDone/1
  Constant1/1 -> Product/1
  Index Vector/1 -> Product/2
  Product/1 -> signal/1
  Logical Operator3/1 -> Logical Operator4/2
  sysID_isDone/1 -> Logical Operator3/1  "isDone"
  TVC_rz_delay/1 -> Logical Operator4/1
  Enable/1 -> TVC_rz_delay/1  "isEnable"
  isTurnOn/1 -> Logical Operator1/1  "isTurnOn"
  Logical Operator4/1 -> Logical Operator1/2  "enableSignal"
  Logical Operator1/1 -> Pause Counter/Enable

== system Copy_of_NDI/F-16 Vehicle Systems Model/sysID_Onboard_Excitation_System/signal generator2 ==
  note: ROM記憶體的指標(Pointer)
  note: 唯讀記憶體，裡面存放波形
  isTurnOn : Inport
  Enable : Inport  Port=2
  sysID_isDone : Inport  Port=3
  Constant1 : Constant  Value=sysID_OBES.TVC_ly.amplitude
  Index Vector : MultiPortSwitch  Inputs=1  SaturateOnIntegerOverflow=off  InputSameDT=off
  Logical Operator1 : Logic  AllPortsSameDT=off  OutDataTypeStr=boolean
  Logical Operator3 : Logic  Operator=NOT  AllPortsSameDT=off  OutDataTypeStr=boolean
  Logical Operator4 : Logic  AllPortsSameDT=off  OutDataTypeStr=boolean
  Pause Counter : Subsystem  TreatAsAtomicUnit=on
  Product : Product
  ROM : Constant  Value=sysID_OBES.TVC_ly.wave
  TVC_ly_delay : Delay  DelayLength=sysID_OBES.TVC_ly.delay/sysID_OBES.Ts  SampleTime=sysID_OBES.Ts
  signal : Outport  OutputWhenDisabled=reset  InitialOutput=0
  isDone : Outport  Port=2
  wires:
  ROM/1 -> Index Vector/2
  Pause Counter/1(CountValue) -> Index Vector/1  "Pointer"
  Pause Counter/2(isCountDone) -> isDone/1
  Constant1/1 -> Product/1
  Index Vector/1 -> Product/2
  Product/1 -> signal/1
  Logical Operator3/1 -> Logical Operator4/2
  sysID_isDone/1 -> Logical Operator3/1  "isDone"
  TVC_ly_delay/1 -> Logical Operator4/1
  Enable/1 -> TVC_ly_delay/1  "isEnable"
  isTurnOn/1 -> Logical Operator1/1  "isTurnOn"
  Logical Operator4/1 -> Logical Operator1/2  "enableSignal"
  Logical Operator1/1 -> Pause Counter/Enable

== system Copy_of_NDI/F-16 Vehicle Systems Model/sysID_Onboard_Excitation_System/signal generator3 ==
  note: ROM記憶體的指標(Pointer)
  note: 唯讀記憶體，裡面存放波形
  isTurnOn : Inport
  Enable : Inport  Port=2
  sysID_isDone : Inport  Port=3
  Constant1 : Constant  Value=sysID_OBES.TVC_lz.amplitude
  Index Vector : MultiPortSwitch  Inputs=1  SaturateOnIntegerOverflow=off  InputSameDT=off
  Logical Operator1 : Logic  AllPortsSameDT=off  OutDataTypeStr=boolean
  Logical Operator3 : Logic  Operator=NOT  AllPortsSameDT=off  OutDataTypeStr=boolean
  Logical Operator4 : Logic  AllPortsSameDT=off  OutDataTypeStr=boolean
  Pause Counter : Subsystem  TreatAsAtomicUnit=on
  Product : Product
  ROM : Constant  Value=sysID_OBES.TVC_lz.wave
  TVC_lz_delay : Delay  DelayLength=sysID_OBES.TVC_lz.delay/sysID_OBES.Ts  SampleTime=sysID_OBES.Ts
  signal : Outport  OutputWhenDisabled=reset  InitialOutput=0
  isDone : Outport  Port=2
  wires:
  ROM/1 -> Index Vector/2
  Pause Counter/1(CountValue) -> Index Vector/1  "Pointer"
  Pause Counter/2(isCountDone) -> isDone/1
  Constant1/1 -> Product/1
  Index Vector/1 -> Product/2
  Product/1 -> signal/1
  Logical Operator3/1 -> Logical Operator4/2
  sysID_isDone/1 -> Logical Operator3/1  "isDone"
  TVC_lz_delay/1 -> Logical Operator4/1
  Enable/1 -> TVC_lz_delay/1  "isEnable"
  isTurnOn/1 -> Logical Operator1/1  "isTurnOn"
  Logical Operator4/1 -> Logical Operator1/2  "enableSignal"
  Logical Operator1/1 -> Pause Counter/Enable

== system Copy_of_NDI/F-16 Vehicle Systems Model/sysID_Onboard_Excitation_System/signal generator4 ==
  note: ROM記憶體的指標(Pointer)
  note: 唯讀記憶體，裡面存放波形
  isTurnOn : Inport
  Enable : Inport  Port=2
  sysID_isDone : Inport  Port=3
  Constant1 : Constant  Value=sysID_OBES.right_aileron.amplitude
  Index Vector : MultiPortSwitch  Inputs=1  SaturateOnIntegerOverflow=off  InputSameDT=off
  Logical Operator1 : Logic  AllPortsSameDT=off  OutDataTypeStr=boolean
  Logical Operator3 : Logic  Operator=NOT  AllPortsSameDT=off  OutDataTypeStr=boolean
  Logical Operator4 : Logic  AllPortsSameDT=off  OutDataTypeStr=boolean
  Pause Counter : Subsystem  TreatAsAtomicUnit=on
  Product : Product
  ROM : Constant  Value=sysID_OBES.right_aileron.wave
  right_aileron_delay : Delay  DelayLength=sysID_OBES.right_aileron.delay/sysID_OBES.Ts  SampleTime=sysID_OBES.Ts
  signal : Outport  OutputWhenDisabled=reset  InitialOutput=0
  isDone : Outport  Port=2
  wires:
  ROM/1 -> Index Vector/2
  Pause Counter/1(CountValue) -> Index Vector/1  "Pointer"
  Pause Counter/2(isCountDone) -> isDone/1
  Constant1/1 -> Product/1
  Index Vector/1 -> Product/2
  Product/1 -> signal/1
  Logical Operator3/1 -> Logical Operator4/2
  sysID_isDone/1 -> Logical Operator3/1  "isDone"
  right_aileron_delay/1 -> Logical Operator4/1
  Enable/1 -> right_aileron_delay/1  "isEnable"
  isTurnOn/1 -> Logical Operator1/1  "isTurnOn"
  Logical Operator4/1 -> Logical Operator1/2  "enableSignal"
  Logical Operator1/1 -> Pause Counter/Enable

== system Copy_of_NDI/F-16 Vehicle Systems Model/sysID_Onboard_Excitation_System/signal generator5 ==
  note: ROM記憶體的指標(Pointer)
  note: 唯讀記憶體，裡面存放波形
  isTurnOn : Inport
  Enable : Inport  Port=2
  sysID_isDone : Inport  Port=3
  Constant1 : Constant  Value=sysID_OBES.left_aileron.amplitude
  Index Vector : MultiPortSwitch  Inputs=1  SaturateOnIntegerOverflow=off  InputSameDT=off
  Logical Operator1 : Logic  AllPortsSameDT=off  OutDataTypeStr=boolean
  Logical Operator3 : Logic  Operator=NOT  AllPortsSameDT=off  OutDataTypeStr=boolean
  Logical Operator4 : Logic  AllPortsSameDT=off  OutDataTypeStr=boolean
  Pause Counter : Subsystem  TreatAsAtomicUnit=on
  Product : Product
  ROM : Constant  Value=sysID_OBES.left_aileron.wave
  left_aileron_delay : Delay  DelayLength=sysID_OBES.left_aileron.delay/sysID_OBES.Ts  SampleTime=sysID_OBES.Ts
  signal : Outport  OutputWhenDisabled=reset  InitialOutput=0
  isDone : Outport  Port=2
  wires:
  ROM/1 -> Index Vector/2
  Pause Counter/1(CountValue) -> Index Vector/1  "Pointer"
  Pause Counter/2(isCountDone) -> isDone/1
  Constant1/1 -> Product/1
  Index Vector/1 -> Product/2
  Product/1 -> signal/1
  Logical Operator3/1 -> Logical Operator4/2
  sysID_isDone/1 -> Logical Operator3/1  "isDone"
  left_aileron_delay/1 -> Logical Operator4/1
  Enable/1 -> left_aileron_delay/1  "isEnable"
  isTurnOn/1 -> Logical Operator1/1  "isTurnOn"
  Logical Operator4/1 -> Logical Operator1/2  "enableSignal"
  Logical Operator1/1 -> Pause Counter/Enable

== system Copy_of_NDI/F-16 Vehicle Systems Model/sysID_Onboard_Excitation_System/signal generator6 ==
  note: ROM記憶體的指標(Pointer)
  note: 唯讀記憶體，裡面存放波形
  isTurnOn : Inport
  Enable : Inport  Port=2
  sysID_isDone : Inport  Port=3
  Constant1 : Constant  Value=sysID_OBES.right_elevator.amplitude
  Index Vector : MultiPortSwitch  Inputs=1  SaturateOnIntegerOverflow=off  InputSameDT=off
  Logical Operator1 : Logic  AllPortsSameDT=off  OutDataTypeStr=boolean
  Logical Operator3 : Logic  Operator=NOT  AllPortsSameDT=off  OutDataTypeStr=boolean
  Logical Operator4 : Logic  AllPortsSameDT=off  OutDataTypeStr=boolean
  Pause Counter : Subsystem  TreatAsAtomicUnit=on
  Product : Product
  ROM : Constant  Value=sysID_OBES.right_elevator.wave
  right_elevator_delay : Delay  DelayLength=sysID_OBES.right_elevator.delay/sysID_OBES.Ts  SampleTime=sysID_OBES.Ts
  signal : Outport  OutputWhenDisabled=reset  InitialOutput=0
  isDone : Outport  Port=2
  wires:
  ROM/1 -> Index Vector/2
  Pause Counter/1(CountValue) -> Index Vector/1  "Pointer"
  Pause Counter/2(isCountDone) -> isDone/1
  Constant1/1 -> Product/1
  Index Vector/1 -> Product/2
  Product/1 -> signal/1
  Logical Operator3/1 -> Logical Operator4/2
  sysID_isDone/1 -> Logical Operator3/1  "isDone"
  right_elevator_delay/1 -> Logical Operator4/1
  Enable/1 -> right_elevator_delay/1  "isEnable"
  isTurnOn/1 -> Logical Operator1/1  "isTurnOn"
  Logical Operator4/1 -> Logical Operator1/2  "enableSignal"
  Logical Operator1/1 -> Pause Counter/Enable

== system Copy_of_NDI/F-16 Vehicle Systems Model/sysID_Onboard_Excitation_System/signal generator7 ==
  note: ROM記憶體的指標(Pointer)
  note: 唯讀記憶體，裡面存放波形
  isTurnOn : Inport
  Enable : Inport  Port=2
  sysID_isDone : Inport  Port=3
  Constant1 : Constant  Value=sysID_OBES.left_elevator.amplitude
  Index Vector : MultiPortSwitch  Inputs=1  SaturateOnIntegerOverflow=off  InputSameDT=off
  Logical Operator1 : Logic  AllPortsSameDT=off  OutDataTypeStr=boolean
  Logical Operator3 : Logic  Operator=NOT  AllPortsSameDT=off  OutDataTypeStr=boolean
  Logical Operator4 : Logic  AllPortsSameDT=off  OutDataTypeStr=boolean
  Pause Counter : Subsystem  TreatAsAtomicUnit=on
  Product : Product
  ROM : Constant  Value=sysID_OBES.left_elevator.wave
  left_elevator_delay : Delay  DelayLength=sysID_OBES.left_elevator.delay/sysID_OBES.Ts  SampleTime=sysID_OBES.Ts
  signal : Outport  OutputWhenDisabled=reset  InitialOutput=0
  isDone : Outport  Port=2
  wires:
  ROM/1 -> Index Vector/2
  Pause Counter/1(CountValue) -> Index Vector/1  "Pointer"
  Pause Counter/2(isCountDone) -> isDone/1
  Constant1/1 -> Product/1
  Index Vector/1 -> Product/2
  Product/1 -> signal/1
  Logical Operator3/1 -> Logical Operator4/2
  sysID_isDone/1 -> Logical Operator3/1  "isDone"
  left_elevator_delay/1 -> Logical Operator4/1
  Enable/1 -> left_elevator_delay/1  "isEnable"
  isTurnOn/1 -> Logical Operator1/1  "isTurnOn"
  Logical Operator4/1 -> Logical Operator1/2  "enableSignal"
  Logical Operator1/1 -> Pause Counter/Enable

== system Copy_of_NDI/F-16 Vehicle Systems Model/sysID_Onboard_Excitation_System/signal generator8 ==
  note: ROM記憶體的指標(Pointer)
  note: 唯讀記憶體，裡面存放波形
  isTurnOn : Inport
  Enable : Inport  Port=2
  sysID_isDone : Inport  Port=3
  Constant1 : Constant  Value=sysID_OBES.rudder.amplitude
  Index Vector : MultiPortSwitch  Inputs=1  SaturateOnIntegerOverflow=off  InputSameDT=off
  Logical Operator1 : Logic  AllPortsSameDT=off  OutDataTypeStr=boolean
  Logical Operator3 : Logic  Operator=NOT  AllPortsSameDT=off  OutDataTypeStr=boolean
  Logical Operator4 : Logic  AllPortsSameDT=off  OutDataTypeStr=boolean
  Pause Counter : Subsystem  TreatAsAtomicUnit=on
  Product : Product
  ROM : Constant  Value=sysID_OBES.rudder.wave
  rudder_delay : Delay  DelayLength=sysID_OBES.rudder.delay/sysID_OBES.Ts  SampleTime=sysID_OBES.Ts
  signal : Outport  OutputWhenDisabled=reset  InitialOutput=0
  isDone : Outport  Port=2
  wires:
  ROM/1 -> Index Vector/2
  Pause Counter/1(CountValue) -> Index Vector/1  "Pointer"
  Pause Counter/2(isCountDone) -> isDone/1
  Constant1/1 -> Product/1
  Index Vector/1 -> Product/2
  Product/1 -> signal/1
  Logical Operator3/1 -> Logical Operator4/2
  sysID_isDone/1 -> Logical Operator3/1  "isDone"
  rudder_delay/1 -> Logical Operator4/1
  Enable/1 -> rudder_delay/1  "isEnable"
  isTurnOn/1 -> Logical Operator1/1  "isTurnOn"
  Logical Operator4/1 -> Logical Operator1/2  "enableSignal"
  Logical Operator1/1 -> Pause Counter/Enable

== system Copy_of_NDI/F-16 Vehicle Systems Model/μαβ NDI Controller/command matrix ==
  note: $g_2 {\left(x\right)}={\left[\begin{array}{ccc} g_{\mu_p } & g_{\mu_q } & g_{\mu_r } \\ g_{\alpha_p } & g_{\alpha_q } & g_{\alpha_r } \\ g_{\beta_p } & g_{\beta_q } & g_{\beta_r } \end{array}\right]}={\left[\begin{array}{ccc} \mathrm{cos}\alpha \mathrm{sec}\beta & 0 & \mathrm{sin}\alpha \mathrm{sec}\beta \\ -\mathrm{cos}\alpha \mathrm{tan}\beta & 1 & -\mathrm{sin}\alpha \mathrm{tan}\beta \\ \mathrm{sin}\alpha & 0 & -\mathrm{cos}\alpha \end{array}\right]}$
  α : Inport
  β : Inport  Port=2
  (1,1) : Fcn  Expr=1/cos(u(2)) * cos(u(1))
  (1,2) : Constant  Value=0
  (1,3) : Fcn  Expr=1/cos(u(2)) * sin(u(1))
  (2,1) : Fcn  Expr=-tan(u(2)) * cos(u(1))
  (2,2) : Constant
  (2,3) : Fcn  Expr=-tan(u(2)) * sin(u(1))
  (3,1) : Fcn  Expr=sin(u(1))
  (3,2) : Constant  Value=0
  (3,3) : Fcn  Expr=-cos(u(1))
  Create 3x3 Matrix : sharedutil/Create 3x3 Matrix  aMode=aMode
  Mux4 : Mux  Inputs=2
  g2 : Outport  VectorParamsAs1DForOutWhenUnconnected=off
  wires:
  α/1 -> Mux4/1
  β/1 -> Mux4/2
  Mux4/1 -> (3,3)/1, (3,1)/1, (2,3)/1, (1,1)/1, (1,3)/1, (2,1)/1
  Create 3x3 Matrix/1 -> g2/1
  (2,2)/1 -> Create 3x3 Matrix/5
  (2,1)/1 -> Create 3x3 Matrix/4
  (2,3)/1 -> Create 3x3 Matrix/6
  (1,3)/1 -> Create 3x3 Matrix/3
  (3,1)/1 -> Create 3x3 Matrix/7
  (1,2)/1 -> Create 3x3 Matrix/2
  (3,2)/1 -> Create 3x3 Matrix/8
  (1,1)/1 -> Create 3x3 Matrix/1
  (3,3)/1 -> Create 3x3 Matrix/9

== system Copy_of_NDI/F-16 Vehicle Systems Model/μαβ NDI Controller/f2 ==
  note: 有指定port dimensions=3。
      | 否則，雖然可以正常執行程式，
      | 但是t=0會跳出錯誤訊息說下一模塊"attitude NDI"內的矩陣運算的dimensions不一致
  note: mu alpha beta
  note: 11 gravity
  note: 10 T
  note: 9 mass
  note: 8 L
  note: 7 Y
  note: 6 D
  note: 1 Vt alpha beta mu gamma
  note: 11 gravity
  note: 9 mass
  note: 6 Xbar Ybar Zbar
  note: 1 Vinf alpha beta mu gamma
  note: 10 T
  note: 12 f 0 N
  note: 12 f 0 N
  note: 15 chi
  note: 15 chi
  aero V : Inport
  X,Y,Z : Inport  Port=2
  gravity : Inport  Port=3
  Thrust : Inport  Port=4
  LGxyz : Inport  Port=5
  chi : Inport  Port=6
  Add : Sum  Inputs=++++
  Add1 : Sum
  Add2 : Sum
  Drag : Fcn  Expr=-u(6)*cos(u(2))*cos(u(3))-u(7)*sin( u(3) )-u(8)*sin(u(2))*cos(u(3))
  Lift : Fcn  Expr=u(6)*sin(u(2))-u(8)*cos(u(2))
  Mux : Mux  Inputs=3
  Mux1 : Mux  Inputs=9
  Mux2 : Mux  Inputs=2
  Side Force : Fcn  Expr=-u(6)*cos(u(2))*sin(u(3))+u(7)*cos( u(3) )-u(8)*sin(u(2))*sin(u(3))
  f_alpha1 : Fcn  Expr=( -u(8)+u(9)*u(11)*cos(u(5))*cos(u(4))-u(10)*sin(u(2)) ) / ( u(9)*u(1)*cos(u(3)) )
  f_alpha2 : Fcn  Expr=( u(14)*cos(u(5))*cos(u(4))+u(12)*sin(u(15))*sin(u(4))+u(12)*cos(u(15))*cos(u(4))*sin(u(5)) ) / ( u(9)*u(1)*cos(u(3)) )
  f_beta1 : Fcn  Expr=( u(7)*cos(u(3))+u(9)*u(11)*cos(u(5))*sin(u(4))-u(10)*cos(u(2))*sin(u(3)) ) / ( u(9)*u(1) )
  f_beta2 : Fcn  Expr=( u(14)*cos(u(5))*sin(u(4))-u(12)*( cos(u(4))*sin(u(15))-cos(u(15))*sin(u(5))*sin(u(4)) ) / ( u(9)*u(1) ) )
  f_mu1 : Fcn  Expr=u(8)*( tan(u(5))*sin(u(4))+tan(u(3)) ) / ( u(9)*u(1) )
  f_mu2 : Fcn  Expr=(u(7)*tan(u(5))*cos(u(4))*cos(u(3)) -u(9)*u(11)*cos(u(5))*cos(u(4))*tan(u(3)) ) / ( u(9)*u(1) )
  f_mu3 : Fcn  Expr=u(10)*( sin(u(2))*tan(u(5))*sin(u(4)) + sin(u(2))*tan(u(3)) - cos(u(2))*tan(u(5))*cos(u(4))*sin(u(3)) ) / ( u(9)*u(1) )
  f_mu4 : Fcn  Expr="( -u(14)*cos(u(5))*cos(u(4))*tan(u(3))-u(12)*( cos(u(4))*cos(u(15))*sin(u(5))*tan(u(3))+sin(u(15))*tan(u(3))*sin(u(4)) )  ) / ( u(9)*u(1) )"
  m(slugs) : Constant  Value=ac.m
  f2 : Outport  PortDimensions=3  VectorParamsAs1DForOutWhenUnconnected=off
  D : Outport  Port=2  VectorParamsAs1DForOutWhenUnconnected=off
  Y : Outport  Port=3  VectorParamsAs1DForOutWhenUnconnected=off
  L : Outport  Port=4  VectorParamsAs1DForOutWhenUnconnected=off
  wires:
  Mux/1 -> f2/1
  aero V/1 -> Mux1/1, Mux2/1  "Vt, α, β, μ, γ"
  X,Y,Z/1 -> Mux2/2  "Xbar, Ybar, Zbar"
  Mux2/1 -> Lift/1, Drag/1, Side Force/1
  Mux1/1 -> f_beta2/1, f_beta1/1, f_alpha2/1, f_alpha1/1, f_mu4/1, f_mu1/1, f_mu2/1, f_mu3/1
  Drag/1 -> Mux1/2, D/1  "D"
  Side Force/1 -> Mux1/3, Y/1  "Y"
  Lift/1 -> Mux1/4, L/1  "L"
  m(slugs)/1 -> Mux1/5
  Thrust/1 -> Mux1/6  "T"
  gravity/1 -> Mux1/7  "g"
  f_mu2/1 -> Add/2
  f_mu1/1 -> Add/1
  Add/1 -> Mux/1
  f_mu3/1 -> Add/3
  LGxyz/1 -> Mux1/8
  chi/1 -> Mux1/9
  f_alpha1/1 -> Add1/1
  f_alpha2/1 -> Add1/2
  Add1/1 -> Mux/2
  Add2/1 -> Mux/3
  f_beta1/1 -> Add2/1
  f_beta2/1 -> Add2/2
  f_mu4/1 -> Add/4
